simulink model "two_layer_distributed_deadbeat"  (R2024b)
settings: Solver=FixedStepAuto  StartTime=0.0  StopTime=40  FixedStep=d_t  RelTol=1e-3
values from neighbouring files (symbols this model uses):
  A = [1 -0.142320298114 0 0.206852817991 0 0.0985289498747 0 0 0 0.0497793964244 0.2 0.963349840614 ... (100 elements, 10x10)]    [first_layer_done.mat]    (also in make_network.m = [A; A_r]; rand_net_params.mat; second_layer_distributed_tracking_robust.m = evalin('base','A'); second_layer_done.mat)
  amp_n_u_f = 1e-3    (= 0.001)    [second_layer_distributed_design_deadbeat.m]    (also in second_layer_done.mat)
  amp_n_u_s2 = 1e-3    (= 0.001)    [second_layer_distributed_design_deadbeat.m]    (also in second_layer_done.mat)
  amp_n_x = 1e-3    (= 0.001)    [second_layer_distributed_design_deadbeat.m]    (also in second_layer_done.mat)
  B = [0 1 0 0 0 0 0 0 0 0 0 0 ... (50 elements, 10x5)]    [first_layer_done.mat]    (also in make_network.m = blkdiag(B,[0;1]); rand_net_params.mat; second_layer_distributed_tracking_robust.m = evalin('base','B'); second_layer_done.mat)
  d_t = 0.2    [first_layer_done.mat]    (also in make_network.m; rand_net_params.mat; second_layer_distributed_tracking_robust.m = evalin('base','d_t'); second_layer_done.mat)
  K_D_sliced = cell(1,5)    [first_layer_design_deadbeat.m]    (also in first_layer_done.mat = ; second_layer_done.mat = )
  r_vec_1 = 0.2 * [1 1 1 1 1]'    [second_layer_distributed_design_deadbeat.m]    (also in second_layer_done.mat = [0.2 0.2 0.2 0.2 0.2])
  r_vec_2 = -0.2 * [1 1 1 1 1]'    [second_layer_distributed_design_deadbeat.m]    (also in second_layer_done.mat = [-0.2 -0.2 -0.2 -0.2 -0.2])
  x0 = [node_1_0; node_2_0; node_3_0; node_4_0; node_5_0]    [second_layer_distributed_design_deadbeat.m]    (also in second_layer_done.mat = [0.157361843197 0.0811583874151 -0.186506591853 0.0826751712)
undefined symbols (not defined in the file or in its folder): second_layer_distributed_tracking_robust
settings Model: Creator=Andrei  LastModifiedBy=Antonio

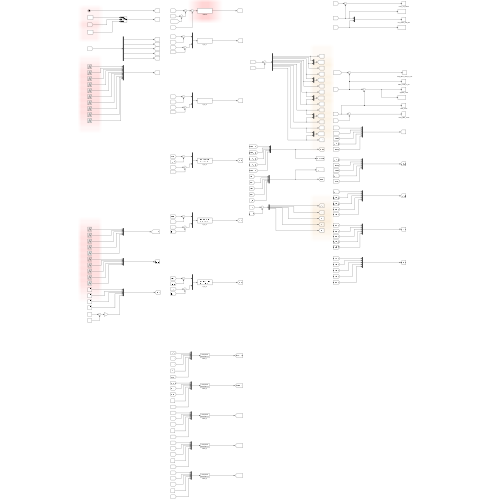
[thumbnail: Simulink's stored preview of the top-level diagram]
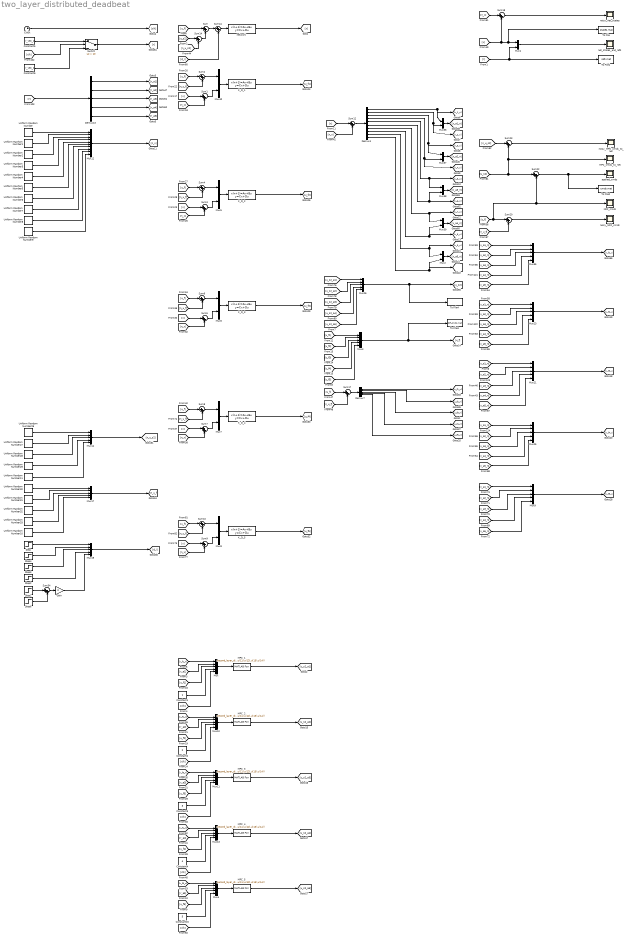
== system two_layer_distributed_deadbeat ==
  Clock : Clock
  Constant1 : Constant  SampleTime=d_t
  Constant15 : Constant  Value=5  SampleTime=d_t
  Constant2 : Constant  Value=2  SampleTime=d_t
  Constant3 : Constant  Value=3  SampleTime=d_t
  Constant4 : Constant  Value=4  SampleTime=d_t
  Constant5 : Constant  Value=r_vec_2  SampleTime=d_t
  Constant6 : Constant  Value=r_vec_1  SampleTime=d_t
  Demux1 : Demux  Outputs=10
  Demux13 : Demux  Outputs=5
  Demux7 : Demux  Outputs=5
  Gain : Gain  Gain=0
  K_D_1 : DiscreteStateSpace  A=K_D_sliced{1}.a  B=K_D_sliced{1}.b  C=K_D_sliced{1}.c  D=K_D_sliced{1}.d  SampleTime=d_t
  K_D_2 : DiscreteStateSpace  A=K_D_sliced{2}.a  B=K_D_sliced{2}.b  C=K_D_sliced{2}.c  D=K_D_sliced{2}.d  SampleTime=d_t
  K_D_3 : DiscreteStateSpace  A=K_D_sliced{3}.a  B=K_D_sliced{3}.b  C=K_D_sliced{3}.c  D=K_D_sliced{3}.d  SampleTime=d_t
  K_D_4 : DiscreteStateSpace  A=K_D_sliced{4}.a  B=K_D_sliced{4}.b  C=K_D_sliced{4}.c  D=K_D_sliced{4}.d  SampleTime=d_t
  K_D_5 : DiscreteStateSpace  A=K_D_sliced{5}.a  B=K_D_sliced{5}.b  C=K_D_sliced{5}.c  D=K_D_sliced{5}.d  SampleTime=d_t
  MPC_{1..5} (5 alike) : MATLABFcn  MATLABFcn=second_layer_distributed_tracking_robust(u(1:10),u(11),u(12),u(13),u(14))  OutputDimensions=1  SampleTime=d_t
  MPC_cmds_to_net : Scope
  Mux{,3..4,9..11,13..14,17,19,21,23,25..26,35} (15 alike) : Mux  Inputs=5
  Mux{1..2,5..8,36..40} (11 alike) : Mux  Inputs=2
  Mux12 : Mux  Inputs=10
  NRF_cmds : Scope
  Step : Step  Time=0  SampleTime=d_t
  Step1 : Step  Time=20  After=0.075  SampleTime=d_t
  Step2 : Step  Time=0  After=0  SampleTime=d_t
  Step3 : Step  Time=0  After=0  SampleTime=d_t
  Step4 : Step  Time=0  After=0  SampleTime=d_t
  Step6 : Step  Time=30  After=-0.075  SampleTime=d_t
  Sum{,1..10,12,14,17..18,20,22..24,34} (20 alike) : Sum  Inputs=|++
  Switch : Switch  Criteria=u2 > Threshold  Threshold=10  SaturateOnIntegerOverflow=off  InputSameDT=off
  To File : ToFile  Filename=states.mat  MatrixName=states  SaveFormat=Timeseries  SampleTime=d_t
  To File1 : ToFile  Filename=refs.mat  MatrixName=refs  SaveFormat=Timeseries  SampleTime=d_t
  To File2 : ToFile  Filename=cmds.mat  MatrixName=cmds  SaveFormat=Timeseries  SampleTime=d_t
  To File3 : ToFile  Filename=NRF_cmds.mat  MatrixName=cmds  SaveFormat=Timeseries  SampleTime=d_t
  To File4 : ToFile  Filename=MPC_cmds.mat  MatrixName=cmds  SaveFormat=Timeseries  SampleTime=d_t
  Uniform Random Number{,1..9} (10 alike) : UniformRandomNumber  Minimum=-amp_n_x  Maximum=amp_n_x  Seed=randi(1000)  SampleTime=d_t
  Uniform Random Number{10,30..33} (5 alike) : UniformRandomNumber  Minimum=-amp_n_u_f  Maximum=amp_n_u_f  Seed=randi(1000)  SampleTime=d_t
  Uniform Random Number{11,26..29} (5 alike) : UniformRandomNumber  Minimum=-amp_n_u_s2  Maximum=amp_n_u_s2  Seed=randi(1000)  SampleTime=d_t
  applied_cmds : Scope
  net_states_and_refs : Scope
  network : DiscreteStateSpace  A=A  B=B  C=eye(size(A))  D=zeros(size(B))  InitialCondition=x0  SampleTime=d_t
  noisy_MPC_cmds_to_net : Scope
  noisy_NRF_cmds : Scope
  noisy_net_states : Scope
  wires:
  [u_f2] -> Mux3/2
  [x] -> Sum12/1
  Sum12/1 -> Demux1/1
  Mux12/1 -> [n_x]
  Uniform Random Number2/1 -> Mux12/3
  Uniform Random Number6/1 -> Mux12/7
  Uniform Random Number3/1 -> Mux12/4
  Demux1/8 -> Mux39/2, [x_8_n]
  K_D_1/1 -> [u_f1]
  [u_f3] -> Mux3/3
  Demux1/4 -> Mux37/2, [x_4_n]
  Uniform Random Number/1 -> Mux12/1
  Demux7/4 -> [u_f4_n]
  Uniform Random Number29/1 -> Mux14/4
  Demux7/2 -> [u_f2_n]
  Demux7/1 -> [u_f1_n]
  [n_u_s2] -> Sum14/2
  [u_f1] -> Mux3/1
  Sum17/1 -> Demux7/1
  Mux14/1 -> [n_u_s2]
  [u_f] -> Sum/1
  Demux1/3 -> Mux37/1, [x_3_n]
  [u_f] -> Sum17/1
  Demux1/7 -> Mux39/1, [x_7_n]
  Uniform Random Number33/1 -> Mux17/4
  Uniform Random Number30/1 -> Mux17/1
  Uniform Random Number31/1 -> Mux17/2
  [n_u_f] -> Sum17/2
  [u_f4] -> Mux3/4
  Mux1/1 -> net_states_and_refs/1
  Sum14/1 -> Sum/2
  network/1 -> [x]
  [n_x] -> Sum12/2
  Uniform Random Number28/1 -> Mux14/3
  [u_s2] -> Sum14/1
  Mux3/1 -> To File3/1, [u_f]
  Uniform Random Number26/1 -> Mux14/1
  Uniform Random Number5/1 -> Mux12/6
  Uniform Random Number32/1 -> Mux17/3
  Uniform Random Number4/1 -> Mux12/5
  Uniform Random Number1/1 -> Mux12/2
  Demux1/2 -> [x_2_n], Mux36/2
  Demux1/1 -> Mux36/1, [x_1_n]
  Demux1/5 -> Mux38/1, [x_5_n]
  Mux17/1 -> [n_u_f]
  [x_f1_n] -> Mux/1
  Uniform Random Number7/1 -> Mux12/8
  Uniform Random Number27/1 -> Mux14/2
  [r] -> Mux1/2, To File1/1
  Clock/1 -> [clk]
  Mux/1 -> MPC_1/1
  [r_a1] -> Mux/2
  [x] -> Sum18/2, To File/1, Mux1/1
  [n_x] -> Sum18/1
  Sum18/1 -> noisy_net_states/1
  [n_u_f] -> Sum20/2
  [u_f] -> Sum22/2, NRF_cmds/1, Sum20/1
  Sum20/1 -> noisy_NRF_cmds/1
  Sum22/1 -> To File2/1, applied_cmds/1
  Sum23/1 -> noisy_MPC_cmds_to_net/1
  [u_s2] -> Sum22/1, Sum23/2, MPC_cmds_to_net/1
  Sum/1 -> Sum24/1
  [d_i] -> Sum24/2
  Sum24/1 -> network/1
  Step/1 -> Mux19/1
  Mux19/1 -> [d_i]
  [u_s2_a3] -> Mux26/3
  [u_s2_a4] -> Mux26/4
  [u_s2_a1] -> Mux26/1
  [u_s2_a2] -> Mux26/2
  Mux26/1 -> To File4/1, [u_s2]
  [r] -> Demux13/1
  Demux13/1 -> [r_a1]
  Demux13/2 -> [r_a2]
  Demux13/3 -> [r_a3]
  Demux13/4 -> [r_a4]
  [x_a1_n] -> Mux35/1
  [x_a2_n] -> Mux35/2
  [x_a3_n] -> Mux35/3
  Mux35/1 -> [x_f1_n]
  Mux36/1 -> [x_a1_n]
  Mux37/1 -> [x_a2_n]
  Mux38/1 -> [x_a3_n]
  Demux1/6 -> Mux38/2, [x_6_n]
  Mux39/1 -> [x_a4_n]
  Constant5/1 -> Switch/1
  Switch/1 -> [r]
  Constant6/1 -> Switch/3
  [clk] -> Switch/2
  Mux40/1 -> K_D_1/1
  Step2/1 -> Mux19/4
  Step6/1 -> Sum34/2
  Step1/1 -> Sum34/1
  Sum34/1 -> Gain/1
  MPC_1/1 -> [u_s2_a1]
  Demux7/3 -> [u_f3_n]
  [u_f1] -> Mux/3
  Constant1/1 -> Mux/4
  [clk] -> Mux/5
  MPC_2/1 -> [u_s2_a2]
  Constant2/1 -> Mux10/4
  Mux10/1 -> MPC_2/1
  [x_f2_n] -> Mux10/1
  [clk] -> Mux10/5
  [r_a2] -> Mux10/2
  [u_f2] -> Mux10/3
  MPC_3/1 -> [u_s2_a3]
  Constant3/1 -> Mux11/4
  Mux11/1 -> MPC_3/1
  [x_f3_n] -> Mux11/1
  [clk] -> Mux11/5
  [r_a3] -> Mux11/2
  [u_f3] -> Mux11/3
  MPC_4/1 -> [u_s2_a4]
  Constant4/1 -> Mux13/4
  Mux13/1 -> MPC_4/1
  [x_f4_n] -> Mux13/1
  [clk] -> Mux13/5
  [r_a4] -> Mux13/2
  [u_f4] -> Mux13/3
  Mux21/1 -> [x_f3_n]
  [x_a1_n] -> Mux21/1
  [x_a3_n] -> Mux21/3
  [x_a4_n] -> Mux21/4
  [x_a2_n] -> Mux23/2
  Mux23/1 -> [x_f2_n]
  [x_a1_n] -> Mux23/1
  [x_a4_n] -> Mux23/4
  [x_a4_n] -> Mux25/4
  [x_a3_n] -> Mux25/3
  Mux25/1 -> [x_f4_n]
  [x_a2_n] -> Mux25/2
  Step4/1 -> Mux19/2
  Gain/1 -> Mux19/5
  [n_u_s2] -> Sum23/1
  Uniform Random Number8/1 -> Mux12/9
  Uniform Random Number9/1 -> Mux12/10
  Demux13/5 -> [r_a5]
  Mux2/1 -> [x_a5_n]
  Demux1/10 -> Mux2/2, [x_10_n]
  Demux1/9 -> Mux2/1, [x_9_n]
  [u_s2_a5] -> Mux26/5
  [u_f5] -> Mux3/5
  Demux7/5 -> [u_f5_n]
  Step3/1 -> Mux19/3
  Uniform Random Number10/1 -> Mux17/5
  Uniform Random Number11/1 -> Mux14/5
  MPC_5/1 -> [u_s2_a5]
  Mux4/1 -> MPC_5/1
  [clk] -> Mux4/5
  [u_f5] -> Mux4/3
  Constant15/1 -> Mux4/4
  [x_f5_n] -> Mux4/1
  [r_a5] -> Mux4/2
  [x_a5_n] -> Mux35/5
  [x_a5_n] -> Mux23/5
  [x_a5_n] -> Mux21/5
  [x_a5_n] -> Mux25/5
  [x_a3_n] -> Mux9/3
  [x_a2_n] -> Mux9/2
  Mux9/1 -> [x_f5_n]
  [x_a4_n] -> Mux9/4
  [x_a5_n] -> Mux9/5
  [x_a1_n] -> Mux9/1
  K_D_2/1 -> [u_f2]
  K_D_3/1 -> [u_f3]
  K_D_4/1 -> [u_f4]
  K_D_5/1 -> [u_f5]
  [x_a4_n] -> Mux35/4
  [x_a3_n] -> Mux23/3
  [x_a2_n] -> Mux21/2
  [x_a1_n] -> Mux25/1
  [n_x] -> Sum1/2
  [x] -> Sum1/1
  Sum1/1 -> Mux40/2
  [n_u_f] -> Sum2/2
  [u_f] -> Sum2/1
  Sum2/1 -> Mux40/1
  Sum4/1 -> Mux5/1
  [u_f] -> Sum4/1
  [x] -> Sum3/1
  Sum3/1 -> Mux5/2
  [n_x] -> Sum3/2
  Mux5/1 -> K_D_2/1
  [n_u_f] -> Sum4/2
  Sum6/1 -> Mux6/1
  [u_f] -> Sum6/1
  [x] -> Sum5/1
  Sum5/1 -> Mux6/2
  [n_x] -> Sum5/2
  Mux6/1 -> K_D_3/1
  [n_u_f] -> Sum6/2
  Sum8/1 -> Mux7/1
  [u_f] -> Sum8/1
  [x] -> Sum7/1
  Sum7/1 -> Mux7/2
  [n_x] -> Sum7/2
  Mux7/1 -> K_D_4/1
  [n_u_f] -> Sum8/2
  Sum10/1 -> Mux8/1
  [u_f] -> Sum10/1
  [x] -> Sum9/1
  Sum9/1 -> Mux8/2
  [n_x] -> Sum9/2
  Mux8/1 -> K_D_5/1
  [n_u_f] -> Sum10/2
